simulink model "INtegrated_Simplified_Batteries_2"  (R2025a)
settings: Solver=ode113  StartTime=0.0  StopTime=20000  FixedStep=0.01  MaxStep=0.1  RelTol=1e-3
libraries: simulink x16, slpidlib x2, spsFirstOrderFilterLib x1
(part 3 of 3)

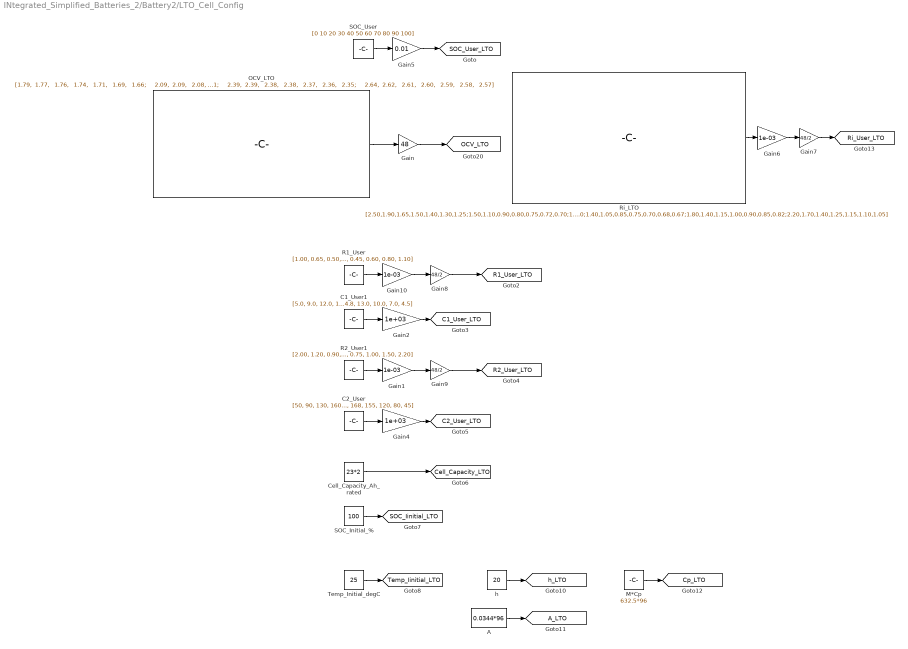
== system INtegrated_Simplified_Batteries_2/Battery2/LTO_Cell_Config ==
  A : Constant  Value=0.0344*96
  C1_User1 : Constant  Value=[5.0, 9.0, 12.0, 14.0, 14.8, 15.0, 14.8, 13.0, 10.0, 7.0, 4.5]
  C2_User : Constant  Value=[50, 90, 130, 160, 168, 170, 168, 155, 120, 80, 45]
  Cell_Capacity_Ah_rated : Constant  Value=23*2
  Gain : Gain  Gain=48
  Gain1 : Gain  Gain=1e-03
  Gain10 : Gain  Gain=1e-03
  Gain2 : Gain  Gain=1e+03
  Gain4 : Gain  Gain=1e+03
  Gain5 : Gain  Gain=0.01
  Gain6 : Gain  Gain=1e-03
  Gain7 : Gain  Gain=48/2
  Gain8 : Gain  Gain=48/2
  Gain9 : Gain  Gain=48/2
  M*Cp : Constant  Value=632.5*96
  OCV_LTO : Constant  Value=|
      | [1.79,  1.77,   1.76,   1.74,   1.71,   1.69,   1.66;
      |     2.09,  2.09,   2.08,   2.07,   2.06,   2.05,   2.04;
      |     2.19,  2.19,   2.18,   2.18,   2.17,   2.16,   2.15;
      |     2.23,  2.23,   2.23,   2.22,   2.22,   2.21,   2.21;
      |     2.25,  2.25,   2.25,   2.24,   2.24,   2.23,   2.23;
      |     2.28,  2.27,   2.27,   2.27,   2.26,   2.26,   2.25;
      |     2.30,  2.29,   2.29,   2.29,   2.28,   2.28,   2.27;
      |     2.32,  2.31,   2.31,   2.31,   2.30,   2.30,   2.29;
      |     2.34,  2.34,   2.34,   2.33,   2.33,   2.32,   2.31;
      |     2.39,  2.39,   2.38,   2.38,   2.37,   2.36,   2.35;
      |     2.64,  2.62,   2.61,   2.60,   2.59,   2.58,   2.57]
  R1_User : Constant  Value=[1.00, 0.65, 0.50, 0.40, 0.37, 0.35, 0.37, 0.45, 0.60, 0.80, 1.10]
  R2_User1 : Constant  Value=[2.00, 1.20, 0.90, 0.70, 0.62, 0.60, 0.62, 0.75, 1.00, 1.50, 2.20]
  Ri_LTO : Constant  Value=[2.50,1.90,1.65,1.50,1.40,1.30,1.25;1.50,1.10,0.90,0.80,0.75,0.72,0.70;1.25,0.95,0.75,0.65,0.60,0.58,0.57;1.10,0.80,0.60,0.52,0.48,0.47,0.46;1.05,0.75,0.55,0.48,0.45,0.44,0.43;1.00,0.70,0.52,0.45,0.42,0.41,0.40;1.05,0.75,0.55,0.48,0.45,0.44,0.43;1.15,0.85,0.65,0.57,0.53,0.51,0.50;1.40,1.05,0.85,0.75,0.70,0.68,0.67;1.80,1.40,1.15,1.00,0.90,0.85,0.82;2.20,1.70,1.40,1.25,1.15,1.10,1.05]
  SOC_Initial_% : Constant  Value=100
  SOC_User : Constant  Value=[0 10 20 30 40 50 60 70 80 90 100]
  Temp_Initial_degC : Constant  Value=25
  h : Constant  Value=20
  tag scope: A_LTO=global, C1_User_LTO=global, C2_User_LTO=global, Cell_Capacity_LTO=global, Cp_LTO=global, OCV_LTO=global, R1_User_LTO=global, R2_User_LTO=global, Ri_User_LTO=global, SOC_Iinitial_LTO=global, SOC_User_LTO=global, Temp_Iinitial_LTO=global, h_LTO=global
  wires:
  OCV_LTO/1 -> Gain/1
  SOC_User/1 -> Gain5/1
  R1_User/1 -> Gain10/1
  Gain10/1 -> Gain8/1
  C1_User1/1 -> Gain2/1
  Gain2/1 -> [C1_User_LTO]
  R2_User1/1 -> Gain1/1
  Gain1/1 -> Gain9/1
  Gain4/1 -> [C2_User_LTO]
  C2_User/1 -> Gain4/1
  Cell_Capacity_Ah_rated/1 -> [Cell_Capacity_LTO]
  SOC_Initial_%/1 -> [SOC_Iinitial_LTO]
  Gain5/1 -> [SOC_User_LTO]
  Temp_Initial_degC/1 -> [Temp_Iinitial_LTO]
  h/1 -> [h_LTO]
  A/1 -> [A_LTO]
  M*Cp/1 -> [Cp_LTO]
  Gain6/1 -> Gain7/1
  Ri_LTO/1 -> Gain6/1
  Gain/1 -> [OCV_LTO]
  Gain7/1 -> [Ri_User_LTO]
  Gain8/1 -> [R1_User_LTO]
  Gain9/1 -> [R2_User_LTO]

== system INtegrated_Simplified_Batteries_2/Battery2/Module2 ==
  Module_Current : Inport
  SubModule_1 : Subsystem
  Module_Voltage : Outport
  Module_avg_Temp : Outport  Port=2
  wires:
  SubModule_1/2(SubModule_avg_temp) -> Module_avg_Temp/1
  [Module_Current] -> SubModule_1/1(Module_Current)
  SubModule_1/1(SubModule_Voltage) -> Module_Voltage/1
  Module_Current/1 -> [Module_Current]

== system INtegrated_Simplified_Batteries_2/Battery2/SOCEstimator ==
  SOC_Initial : Inport
  Pack_Capacity : Inport  Port=2
  Current : Inport  Port=3
  SOCEstimator : Subsystem
  SOC : Outport
  wires:
  SOCEstimator/1(SOC) -> SOC/1
  SOC_Initial/1 -> SOCEstimator/1(SOC_Initial)
  Current/1 -> SOCEstimator/2(Current)
  Pack_Capacity/1 -> SOCEstimator/3(CellCapacity)

== system INtegrated_Simplified_Batteries_2/Observations/Battery1 Operation ==
  Battery1_Voltage : Inport
  Battery1_Current : Inport  Port=2
  Battery1_DischargeCurrLim : Inport  Port=3
  Battery1_ChargeCurrLim : Inport  Port=4
  Battery1_SOC : Inport  Port=5
  Battery1_Temperature : Inport  Port=6
  Battery1_Power : Inport  Port=7
  Battery1_Currents,Current_Limits&SOC : Scope  NumInputPorts=2
      settings: ActiveDisplayYMinimum=-282.10404867069661  ActiveDisplayYMaximum=307.35303677527855  DataLoggingVariableName=ScopeData2
  Battery1_Power&Temperature : Scope  NumInputPorts=2
      settings: ActiveDisplayYMinimum=22.791711351497295  ActiveDisplayYMaximum=44.874597836524366  DataLoggingVariableName=ScopeData3
  Battery1_Voltage&SOC : Scope  NumInputPorts=2
      settings: ActiveDisplayYMinimum=-1  ActiveDisplayYMaximum=1
  Mux : Mux  Inputs=3
  wires:
  Battery1_Voltage/1 -> Battery1_Voltage&SOC/1
  Battery1_SOC/1 -> Battery1_Voltage&SOC/2, Battery1_Currents,Current_Limits&SOC/2
  Mux/1 -> Battery1_Currents,Current_Limits&SOC/1
  Battery1_Current/1 -> Mux/1
  Battery1_DischargeCurrLim/1 -> Mux/2
  Battery1_ChargeCurrLim/1 -> Mux/3
  Battery1_Temperature/1 -> Battery1_Power&Temperature/1
  Battery1_Power/1 -> Battery1_Power&Temperature/2

== system INtegrated_Simplified_Batteries_2/Observations/Battery2 Operation ==
  Battery2_Voltage : Inport
  Battery2_Current : Inport  Port=2
  Battery2_DischargeCurrLim : Inport  Port=3
  Battery2_ChargeCurrLim : Inport  Port=4
  Battery2_SOC : Inport  Port=5
  Battery2_Temperature : Inport  Port=6
  Battery2_Power : Inport  Port=7
  Battery2_Currents,Current_Limits&SOC : Scope  NumInputPorts=2
      settings: ActiveDisplayYMinimum=-1129.3572740653772  ActiveDisplayYMaximum=1109.43488760312  DataLoggingVariableName=ScopeData2
  Battery2_Power&Temperature : Scope  NumInputPorts=2
      settings: ActiveDisplayYMinimum=22.713194675868088  ActiveDisplayYMaximum=45.581247917187227  DataLoggingVariableName=ScopeData3
  Battery2_Voltage&SOC : Scope  NumInputPorts=2
      settings: ActiveDisplayYMinimum=-1  ActiveDisplayYMaximum=1
  Mux : Mux  Inputs=3
  wires:
  Battery2_SOC/1 -> Battery2_Voltage&SOC/2, Battery2_Currents,Current_Limits&SOC/2
  Battery2_Voltage/1 -> Battery2_Voltage&SOC/1
  Battery2_ChargeCurrLim/1 -> Mux/3
  Battery2_Temperature/1 -> Battery2_Power&Temperature/1
  Battery2_Power/1 -> Battery2_Power&Temperature/2
  Battery2_DischargeCurrLim/1 -> Mux/2
  Battery2_Current/1 -> Mux/1
  Mux/1 -> Battery2_Currents,Current_Limits&SOC/1

== system INtegrated_Simplified_Batteries_2/Observations/DAB & Load Splitter Operation ==
  DAB_HighSideCurrentRef : Inport
  DAB_HighSideCurrent : Inport  Port=2
  DAB_PowerTransfer : Inport  Port=3
  Battery1_Current : Inport  Port=4
  Battery2_Current : Inport  Port=5
  Total_Current : Inport  Port=6
  Currents : Scope  NumInputPorts=2
      settings: ActiveDisplayYMinimum=-302.947845806585  ActiveDisplayYMaximum=379.10772170406915  DataLoggingVariableName=ScopeData6
  DAB_HighSideCurr : Scope  NumInputPorts=2
      settings: ActiveDisplayYMinimum=-1  ActiveDisplayYMaximum=1  DataLoggingVariableName=ScopeData4
  DAB_Power : Scope
      settings: ActiveDisplayYMinimum=-1  ActiveDisplayYMaximum=1  DataLoggingVariableName=ScopeData5
  Mux : Mux  Inputs=3
  wires:
  DAB_PowerTransfer/1 -> DAB_Power/1
  DAB_HighSideCurrent/1 -> DAB_HighSideCurr/2, Mux/2
  Battery1_Current/1 -> Mux/1
  Total_Current/1 -> Mux/3
  DAB_HighSideCurrentRef/1 -> DAB_HighSideCurr/1
  Mux/1 -> Currents/1
  Battery2_Current/1 -> Currents/2

== system INtegrated_Simplified_Batteries_2/Observations/System Operation ==
  RPM_request : Inport
  RPM_Actual : Inport  Port=2
  Vehicle_Speed : Inport  Port=3
  Electrical_Power : Inport  Port=4
  Mechanical_Power : Inport  Port=5
  System_Efficiency : Inport  Port=6
  Driveline_Torque_Request : Inport  Port=7
  Driveline_Torque : Inport  Port=8
  Avauilable_Motor_Torque : Inport  Port=9
  Vehicle_Acceleration : Inport  Port=10
  Motor_torque_Actual : Inport  Port=11
  Distance : Inport  Port=12
  Distance_Travelled : Display
  Mux : Mux  Inputs=2
  Mux1 : Mux  Inputs=2
  Mux2 : Mux  Inputs=2
  Power&Efficiency : Scope  NumInputPorts=2
      settings: ActiveDisplayYMinimum=-244.19267618677512  ActiveDisplayYMaximum=191.67830084577145  DataLoggingVariableName=ScopeData8
  RPM_Requested&Actual : Scope  NumInputPorts=2
      settings: ActiveDisplayYMinimum=-2374.9999999999995  ActiveDisplayYMaximum=21375  DataLoggingVariableName=ScopeData7
  Requested&Actual_Torques : Scope  NumInputPorts=3
      settings: ActiveDisplayYMinimum=-499.22287325827932  ActiveDisplayYMaximum=499.91365258425321  DataLoggingVariableName=ScopeData9
  VehicleSpeed&Acceleration : Scope  NumInputPorts=2
      settings: ActiveDisplayYMinimum=-1  ActiveDisplayYMaximum=1  DataLoggingVariableName=ScopeData10
  wires:
  RPM_request/1 -> Mux2/1
  RPM_Actual/1 -> Mux2/2
  Electrical_Power/1 -> Mux/1
  Mechanical_Power/1 -> Mux/2
  System_Efficiency/1 -> Power&Efficiency/2
  Mux/1 -> Power&Efficiency/1
  Mux1/1 -> Requested&Actual_Torques/1
  Driveline_Torque_Request/1 -> Mux1/1
  Driveline_Torque/1 -> Mux1/2
  Avauilable_Motor_Torque/1 -> Requested&Actual_Torques/2
  Vehicle_Speed/1 -> RPM_Requested&Actual/2, VehicleSpeed&Acceleration/1
  Mux2/1 -> RPM_Requested&Actual/1
  Vehicle_Acceleration/1 -> VehicleSpeed&Acceleration/2
  Motor_torque_Actual/1 -> Requested&Actual_Torques/3
  Distance/1 -> Distance_Travelled/1

== system INtegrated_Simplified_Batteries_2/Battery1/Module3/SubModule_1 ==
  Module_Current : Inport
  Cell1 : Subsystem
  SubModule_Voltage : Outport
  SubModule_avg_temp : Outport  Port=2
  wires:
  Cell1/2(Cell_temp) -> SubModule_avg_temp/1
  Cell1/1(Cell_Voltage) -> SubModule_Voltage/1
  [Cell_Current] -> Cell1/1(Cell_Current)
  Module_Current/1 -> [Cell_Current]

== system INtegrated_Simplified_Batteries_2/Battery1/SOCEstimator/SOCEstimator ==
  SOC_Initial : Inport
  Current : Inport  Port=2
  CellCapacity : Inport  Port=3
  Add1 : Sum  Inputs=+-
  Constant : Constant  Value=100  SampleTime=-1
  Constant1 : Constant  Value=3600  SampleTime=-1
  Delay : Delay  DelayLength=1  InitialConditionSource=Input port
      settings: InputPortMap=u0,p4
  Divide : Product  Inputs=*//
  Divide1 : Product  Inputs=*/
  Integrator : Integrator
  Rate Transition : RateTransition
  Saturation1 : Saturate  UpperLimit=1  LowerLimit=0
  SOC : Outport
  wires:
  Add1/1 -> Saturation1/1
  Constant/1 -> Divide1/2
  Divide1/1 -> Delay/2, Add1/1
  Divide/1 -> Add1/2
  Saturation1/1 -> Delay/1
  SOC_Initial/1 -> Divide1/1
  Current/1 -> Integrator/1
  Delay/1 -> Rate Transition/1
  CellCapacity/1 -> Divide/2
  Constant1/1 -> Divide/3
  Integrator/1 -> Divide/1
  Rate Transition/1 -> SOC/1

== system INtegrated_Simplified_Batteries_2/Battery2/Module2/SubModule_1 ==
  Module_Current : Inport
  Cell1 : Subsystem
  SubModule_Voltage : Outport
  SubModule_avg_temp : Outport  Port=2
  wires:
  Cell1/1(Cell_Voltage) -> SubModule_Voltage/1
  [Cell_Current] -> Cell1/1(Cell_Current)
  Module_Current/1 -> [Cell_Current]
  Cell1/2(Cell_temp) -> SubModule_avg_temp/1

== system INtegrated_Simplified_Batteries_2/Battery2/SOCEstimator/SOCEstimator ==
  SOC_Initial : Inport
  Current : Inport  Port=2
  CellCapacity : Inport  Port=3
  Add1 : Sum  Inputs=+-
  Constant : Constant  Value=100  SampleTime=-1
  Constant1 : Constant  Value=3600  SampleTime=-1
  Delay : Delay  DelayLength=1  InitialConditionSource=Input port
      settings: InputPortMap=u0,p4
  Divide : Product  Inputs=*//
  Divide1 : Product  Inputs=*/
  Integrator : Integrator
  Rate Transition : RateTransition
  Saturation1 : Saturate  UpperLimit=1  LowerLimit=0
  SOC : Outport
  wires:
  Add1/1 -> Saturation1/1
  Constant/1 -> Divide1/2
  Divide1/1 -> Delay/2, Add1/1
  Divide/1 -> Add1/2
  Saturation1/1 -> Delay/1
  SOC_Initial/1 -> Divide1/1
  Current/1 -> Integrator/1
  Delay/1 -> Rate Transition/1
  CellCapacity/1 -> Divide/2
  Constant1/1 -> Divide/3
  Integrator/1 -> Divide/1
  Rate Transition/1 -> SOC/1

== system INtegrated_Simplified_Batteries_2/Battery1/Module3/SubModule_1/Cell1 ==
  Cell_Current : Inport
  2RC : Subsystem
  Add : Sum  Inputs=---+
  Lookup Table Dynamic2 : simulink/Lookup Tables/Lookup Table Dynamic  LookUpMeth=Interpolation-Use End Values  OutDataType=fixdt('double')  OutScaling=[]  OutputDataTypeScalingMode=Specify via dialog  OutDataTypeStr=fixdt('double')  DoSatur=off
  Product : Product
  Redution_factor : Constant  Value=[0.8 0.85 0.88 0.95 1 0.98 0.95]
  SOCEstimator : Subsystem  TreatAsAtomicUnit=on
  SOC_Mapping : Subsystem
  Scope : Scope
      settings: DataLoggingSaveFormat=Array
  Scope1 : Scope
      settings: DataLoggingVariableName=ScopeData2  DataLoggingSaveFormat=Array
  Scope2 : Scope
      settings: DataLoggingSaveFormat=Array
  Subsystem : Subsystem
  Temp : Constant  Value=[0 10 20 30 40 50 60]
  Cell_Voltage : Outport
  Cell_temp : Outport  Port=2
  wires:
  Redution_factor/1 -> Lookup Table Dynamic2/3
  Temp/1 -> Lookup Table Dynamic2/2
  Lookup Table Dynamic2/1 -> Product/2
  Product/1 -> SOCEstimator/3(Cell_Capacity)
  Subsystem/1(Temp_Cell) -> Cell_temp/1, Lookup Table Dynamic2/1, SOC_Mapping/2(Cell_Temp), Scope1/1
  SOC_Mapping/6(OCV) -> Add/4
  [SOC_Iinitial] -> SOCEstimator/1(SOC_Initial)
  SOC_Mapping/4(R2) -> 2RC/5(R2)
  SOC_Mapping/5(C2) -> 2RC/6(C2)
  [Cell_Capacity] -> Product/1
  SOC_Mapping/2(R1) -> 2RC/3(R1)
  Cell_Current/1 -> SOCEstimator/2(Current), 2RC/1(Current), Subsystem/1(Cell_Current)
  2RC/3(Vi) -> Add/3
  2RC/1(V1) -> Add/1
  SOC_Mapping/1(Ri) -> 2RC/2(Ri), Subsystem/2(Ri)
  Add/1 -> Cell_Voltage/1, Scope2/1
  SOCEstimator/1(SOC) -> Scope/1, SOC_Mapping/1(SOC)
  SOC_Mapping/3(C1) -> 2RC/4(C1)
  2RC/2(V2) -> Add/2

== system INtegrated_Simplified_Batteries_2/Battery2/Module2/SubModule_1/Cell1 ==
  Cell_Current : Inport
  2RC : Subsystem
  Add : Sum  Inputs=---+
  Lookup Table Dynamic2 : simulink/Lookup Tables/Lookup Table Dynamic  LookUpMeth=Interpolation-Use End Values  OutDataType=fixdt('double')  OutScaling=[]  OutputDataTypeScalingMode=Specify via dialog  OutDataTypeStr=fixdt('double')  DoSatur=off
  Product : Product
  Redution_factor : Constant  Value=[0.8 0.85 0.88 0.95 1 0.98 0.95]
  SOCEstimator : Subsystem  TreatAsAtomicUnit=on
  SOC_Mapping : Subsystem
  Scope : Scope
      settings: DataLoggingSaveFormat=Array
  Scope1 : Scope
      settings: DataLoggingVariableName=ScopeData2  DataLoggingSaveFormat=Array
  Scope2 : Scope
      settings: DataLoggingSaveFormat=Array
  Subsystem : Subsystem
  Temp : Constant  Value=[0 10 20 30 40 50 60]
  Cell_Voltage : Outport
  Cell_temp : Outport  Port=2
  wires:
  Redution_factor/1 -> Lookup Table Dynamic2/3
  Temp/1 -> Lookup Table Dynamic2/2
  Lookup Table Dynamic2/1 -> Product/2
  Product/1 -> SOCEstimator/3(Cell_Capacity)
  Subsystem/1(Temp_Cell) -> Cell_temp/1, Lookup Table Dynamic2/1, SOC_Mapping/2(Cell_Temp), Scope1/1
  SOC_Mapping/6(OCV) -> Add/4
  [SOC_Iinitial_LTO] -> SOCEstimator/1(SOC_Initial)
  SOC_Mapping/4(R2) -> 2RC/5(R2)
  SOC_Mapping/5(C2) -> 2RC/6(C2)
  [Cell_Capacity_LTO] -> Product/1
  SOC_Mapping/2(R1) -> 2RC/3(R1)
  Cell_Current/1 -> SOCEstimator/2(Current), 2RC/1(Current), Subsystem/1(Cell_Current)
  2RC/3(Vi) -> Add/3
  2RC/1(V1) -> Add/1
  SOC_Mapping/1(Ri) -> 2RC/2(Ri), Subsystem/2(Ri)
  Add/1 -> Cell_Voltage/1, Scope2/1
  SOCEstimator/1(SOC) -> Scope/1, SOC_Mapping/1(SOC)
  SOC_Mapping/3(C1) -> 2RC/4(C1)
  2RC/2(V2) -> Add/2

== system INtegrated_Simplified_Batteries_2/Battery1/Module3/SubModule_1/Cell1/2RC ==
  Current : Inport
  Ri : Inport  Port=2
  R1 : Inport  Port=3
  C1 : Inport  Port=4
  R2 : Inport  Port=5
  C2 : Inport  Port=6
  RC1 : Subsystem
  RC2 : Subsystem
  Rint : Subsystem
  V1 : Outport
  V2 : Outport  Port=2
  Vi : Outport  Port=3
  wires:
  Ri/1 -> Rint/2(R)
  C2/1 -> RC2/3(C)
  RC2/1(V) -> V2/1
  RC1/1(V) -> V1/1
  R2/1 -> RC2/2(R)
  C1/1 -> RC1/3(C)
  Rint/1(V) -> Vi/1
  R1/1 -> RC1/2(R)
  Current/1 -> RC2/1(Current), RC1/1(Current), Rint/1(Current)

== system INtegrated_Simplified_Batteries_2/Battery1/Module3/SubModule_1/Cell1/SOCEstimator ==
  SOC_Initial : Inport
  Current : Inport  Port=2
  Cell_Capacity : Inport  Port=3
  SOCEstimator : Subsystem
  SOC : Outport
  wires:
  Cell_Capacity/1 -> SOCEstimator/3(CellCapacity)
  Current/1 -> SOCEstimator/2(Current)
  SOC_Initial/1 -> SOCEstimator/1(SOC_Initial)
  SOCEstimator/1(SOC) -> SOC/1

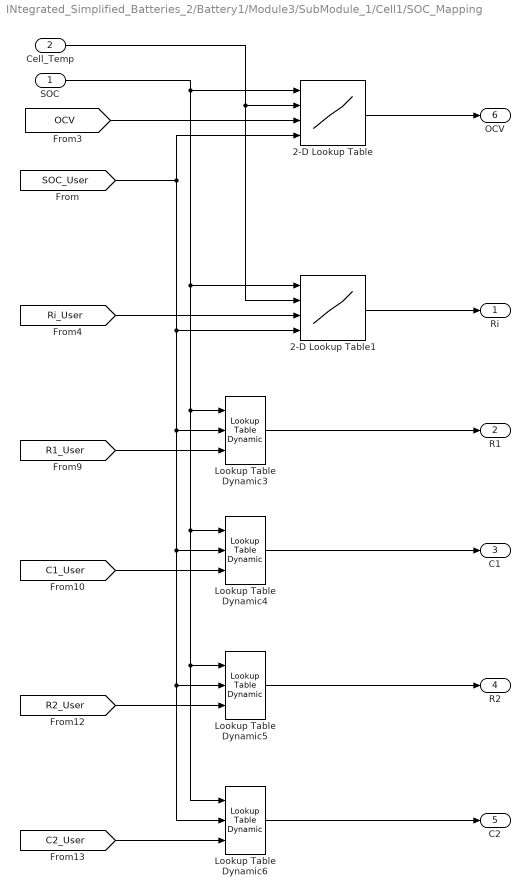
== system INtegrated_Simplified_Batteries_2/Battery1/Module3/SubModule_1/Cell1/SOC_Mapping ==
  SOC : Inport
  Cell_Temp : Inport  Port=2
  2-D Lookup Table : Lookup_n-D  LookupTableObject=''  BreakpointsForDimension1Source=Input port  BreakpointsForDimension1=[0 0.1 0.2 0.3 0.4 0.5 0.6 0.7 0.8 0.9 1]  BreakpointsForDimension2=[0 10 20 30 40 50 60]  BreakpointsForDimension1FirstPoint=10  BreakpointsForDimension2FirstPoint=10  BreakpointsForDimension1Spacing=12  BreakpointsForDimension2Spacing=12  IndexSearchMethod=Evenly spaced points  TableSource=Input port  Table=|  InterpMethod=Akima spline  DiagnosticForOutOfRangeInput=Error  InternalRulePriority=Speed  RndMeth=Simplest
      | [
      |     2.954364, 3.109857, 3.273534, 3.3066, 3.34,    3.3734,  3.20473;
      |     3.122427, 3.286765, 3.459753, 3.4947, 3.53,    3.5653,  3.387035;
      |     3.175499, 3.342631, 3.518559, 3.5541, 3.59,    3.6259,  3.444605;
      |     3.210881, 3.379875, 3.557763, 3.5937, 3.63,    3.6663,  3.482985;
      |     3.237417, 3.407808, 3.587166, 3.6234, 3.66,    3.6966,  3.511777;
      |     3.272799, 3.445052, 3.62637,  3.663,  3.7,     3.737,   3.55015;
      |     3.317026, 3.491066, 3.675375, 3.7125, 3.75,    3.7875,  3.598125;
      |     3.387789, 3.566094, 3.753783, 3.7917, 3.83,    3.8683,  3.674885;
      |     3.467398, 3.649892, 3.841992, 3.8808, 3.92,    3.9592,  3.76124;
      |     3.564697, 3.752313, 3.949803, 3.9897, 4.03,    4.0703,  3.866785;
      |     3.653151, 3.845422, 4.047813, 4.0887, 4.13,    4.1713,  3.962735
      | ]
      settings: InputPortMap=u0,u1,p221,p5
  2-D Lookup Table1 : Lookup_n-D  LookupTableObject=''  BreakpointsForDimension1Source=Input port  BreakpointsForDimension1=[0 0.1 0.2 0.3 0.4 0.5 0.6 0.7 0.8 0.9 1]  BreakpointsForDimension2=[0 10 20 30 40 50 60]  BreakpointsForDimension1FirstPoint=10  BreakpointsForDimension2FirstPoint=10  BreakpointsForDimension1Spacing=12  BreakpointsForDimension2Spacing=12  IndexSearchMethod=Evenly spaced points  TableSource=Input port  Table=|  InterpMethod=Akima spline  DiagnosticForOutOfRangeInput=Error  InternalRulePriority=Speed  RndMeth=Simplest
      | [
      |     2.954364, 3.109857, 3.273534, 3.3066, 3.34,    3.3734,  3.20473;
      |     3.122427, 3.286765, 3.459753, 3.4947, 3.53,    3.5653,  3.387035;
      |     3.175499, 3.342631, 3.518559, 3.5541, 3.59,    3.6259,  3.444605;
      |     3.210881, 3.379875, 3.557763, 3.5937, 3.63,    3.6663,  3.482985;
      |     3.237417, 3.407808, 3.587166, 3.6234, 3.66,    3.6966,  3.511777;
      |     3.272799, 3.445052, 3.62637,  3.663,  3.7,     3.737,   3.55015;
      |     3.317026, 3.491066, 3.675375, 3.7125, 3.75,    3.7875,  3.598125;
      |     3.387789, 3.566094, 3.753783, 3.7917, 3.83,    3.8683,  3.674885;
      |     3.467398, 3.649892, 3.841992, 3.8808, 3.92,    3.9592,  3.76124;
      |     3.564697, 3.752313, 3.949803, 3.9897, 4.03,    4.0703,  3.866785;
      |     3.653151, 3.845422, 4.047813, 4.0887, 4.13,    4.1713,  3.962735
      | ]
      settings: InputPortMap=u0,u1,p221,p5
  Lookup Table Dynamic{3..6} (4 alike) : simulink/Lookup Tables/Lookup Table Dynamic  LookUpMeth=Interpolation-Use End Values  OutDataType=fixdt('double')  OutScaling=[]  OutputDataTypeScalingMode=Specify via dialog  OutDataTypeStr=fixdt('double')  DoSatur=off
  Ri : Outport
  R1 : Outport  Port=2
  C1 : Outport  Port=3
  R2 : Outport  Port=4
  C2 : Outport  Port=5
  OCV : Outport  Port=6
  wires:
  Cell_Temp/1 -> 2-D Lookup Table/2, 2-D Lookup Table1/2
  Lookup Table Dynamic6/1 -> C2/1
  [C2_User] -> Lookup Table Dynamic6/3
  Lookup Table Dynamic5/1 -> R2/1
  [R2_User] -> Lookup Table Dynamic5/3
  Lookup Table Dynamic4/1 -> C1/1
  [C1_User] -> Lookup Table Dynamic4/3
  Lookup Table Dynamic3/1 -> R1/1
  [R1_User] -> Lookup Table Dynamic3/3
  2-D Lookup Table1/1 -> Ri/1
  [Ri_User] -> 2-D Lookup Table1/3
  2-D Lookup Table/1 -> OCV/1
  [OCV] -> 2-D Lookup Table/3
  [SOC_User] -> 2-D Lookup Table1/4, Lookup Table Dynamic3/2, Lookup Table Dynamic4/2, Lookup Table Dynamic5/2, Lookup Table Dynamic6/2, 2-D Lookup Table/4
  SOC/1 -> 2-D Lookup Table/1, 2-D Lookup Table1/1, Lookup Table Dynamic4/1, Lookup Table Dynamic5/1, Lookup Table Dynamic6/1, Lookup Table Dynamic3/1

== system INtegrated_Simplified_Batteries_2/Battery1/Module3/SubModule_1/Cell1/Subsystem ==
  Cell_Current : Inport
  Ri : Inport  Port=2
  Add : Sum  Inputs=+-
  Add1 : Sum  Inputs=-+
  Delay : Delay  DelayLength=1  InitialConditionSource=Input port
      settings: InputPortMap=u0,p4
  Divide : Product  Inputs=*/
  From3 : From  TagVisibility=global
  Integrator : Integrator  InitialConditionSource=external
  Product{,1..3} (4 alike) : Product
  Temp_Cell : Outport
  wires:
  [Cp] -> Divide/2
  Delay/1 -> Add/1
  [Temp_Iinitial] -> Integrator/2, Delay/2
  Divide/1 -> Integrator/1
  Add1/1 -> Divide/1
  Product1/1 -> Add1/2
  Product3/1 -> Add1/1
  Add/1 -> Product3/1
  [Temp_ambient] -> Add/2
  Product2/1 -> Product3/2
  From3/1 -> Product2/2
  [h] -> Product2/1
  Ri/1 -> Product1/2
  Product/1 -> Product1/1
  Cell_Current/1 -> Product/1, Product/2
  Integrator/1 -> Delay/1, Temp_Cell/1

== system INtegrated_Simplified_Batteries_2/Battery2/Module2/SubModule_1/Cell1/2RC ==
  Current : Inport
  Ri : Inport  Port=2
  R1 : Inport  Port=3
  C1 : Inport  Port=4
  R2 : Inport  Port=5
  C2 : Inport  Port=6
  RC1 : Subsystem
  RC2 : Subsystem
  Rint : Subsystem
  V1 : Outport
  V2 : Outport  Port=2
  Vi : Outport  Port=3
  wires:
  Ri/1 -> Rint/2(R)
  C2/1 -> RC2/3(C)
  RC2/1(V) -> V2/1
  RC1/1(V) -> V1/1
  R2/1 -> RC2/2(R)
  C1/1 -> RC1/3(C)
  Rint/1(V) -> Vi/1
  R1/1 -> RC1/2(R)
  Current/1 -> RC2/1(Current), RC1/1(Current), Rint/1(Current)

== system INtegrated_Simplified_Batteries_2/Battery2/Module2/SubModule_1/Cell1/SOCEstimator ==
  SOC_Initial : Inport
  Current : Inport  Port=2
  Cell_Capacity : Inport  Port=3
  SOCEstimator : Subsystem
  SOC : Outport
  wires:
  Cell_Capacity/1 -> SOCEstimator/3(CellCapacity)
  Current/1 -> SOCEstimator/2(Current)
  SOC_Initial/1 -> SOCEstimator/1(SOC_Initial)
  SOCEstimator/1(SOC) -> SOC/1

== system INtegrated_Simplified_Batteries_2/Battery2/Module2/SubModule_1/Cell1/SOC_Mapping ==
  SOC : Inport
  Cell_Temp : Inport  Port=2
  2-D Lookup Table : Lookup_n-D  LookupTableObject=''  BreakpointsForDimension1Source=Input port  BreakpointsForDimension1=[0 0.1 0.2 0.3 0.4 0.5 0.6 0.7 0.8 0.9 1]  BreakpointsForDimension2=[0 10 20 30 40 50 60]  BreakpointsForDimension1FirstPoint=10  BreakpointsForDimension2FirstPoint=10  BreakpointsForDimension1Spacing=12  BreakpointsForDimension2Spacing=12  IndexSearchMethod=Evenly spaced points  TableSource=Input port  Table=|  InterpMethod=Akima spline  DiagnosticForOutOfRangeInput=Error  InternalRulePriority=Speed  RndMeth=Simplest
      | [
      |     2.954364, 3.109857, 3.273534, 3.3066, 3.34,    3.3734,  3.20473;
      |     3.122427, 3.286765, 3.459753, 3.4947, 3.53,    3.5653,  3.387035;
      |     3.175499, 3.342631, 3.518559, 3.5541, 3.59,    3.6259,  3.444605;
      |     3.210881, 3.379875, 3.557763, 3.5937, 3.63,    3.6663,  3.482985;
      |     3.237417, 3.407808, 3.587166, 3.6234, 3.66,    3.6966,  3.511777;
      |     3.272799, 3.445052, 3.62637,  3.663,  3.7,     3.737,   3.55015;
      |     3.317026, 3.491066, 3.675375, 3.7125, 3.75,    3.7875,  3.598125;
      |     3.387789, 3.566094, 3.753783, 3.7917, 3.83,    3.8683,  3.674885;
      |     3.467398, 3.649892, 3.841992, 3.8808, 3.92,    3.9592,  3.76124;
      |     3.564697, 3.752313, 3.949803, 3.9897, 4.03,    4.0703,  3.866785;
      |     3.653151, 3.845422, 4.047813, 4.0887, 4.13,    4.1713,  3.962735
      | ]
      settings: InputPortMap=u0,u1,p221,p5
  2-D Lookup Table1 : Lookup_n-D  LookupTableObject=''  BreakpointsForDimension1Source=Input port  BreakpointsForDimension1=[0 0.1 0.2 0.3 0.4 0.5 0.6 0.7 0.8 0.9 1]  BreakpointsForDimension2=[0 10 20 30 40 50 60]  BreakpointsForDimension1FirstPoint=10  BreakpointsForDimension2FirstPoint=10  BreakpointsForDimension1Spacing=12  BreakpointsForDimension2Spacing=12  IndexSearchMethod=Evenly spaced points  TableSource=Input port  Table=|  InterpMethod=Akima spline  InternalRulePriority=Speed  RndMeth=Simplest
      | [
      |     2.954364, 3.109857, 3.273534, 3.3066, 3.34,    3.3734,  3.20473;
      |     3.122427, 3.286765, 3.459753, 3.4947, 3.53,    3.5653,  3.387035;
      |     3.175499, 3.342631, 3.518559, 3.5541, 3.59,    3.6259,  3.444605;
      |     3.210881, 3.379875, 3.557763, 3.5937, 3.63,    3.6663,  3.482985;
      |     3.237417, 3.407808, 3.587166, 3.6234, 3.66,    3.6966,  3.511777;
      |     3.272799, 3.445052, 3.62637,  3.663,  3.7,     3.737,   3.55015;
      |     3.317026, 3.491066, 3.675375, 3.7125, 3.75,    3.7875,  3.598125;
      |     3.387789, 3.566094, 3.753783, 3.7917, 3.83,    3.8683,  3.674885;
      |     3.467398, 3.649892, 3.841992, 3.8808, 3.92,    3.9592,  3.76124;
      |     3.564697, 3.752313, 3.949803, 3.9897, 4.03,    4.0703,  3.866785;
      |     3.653151, 3.845422, 4.047813, 4.0887, 4.13,    4.1713,  3.962735
      | ]
      settings: InputPortMap=u0,u1,p221,p5
  Lookup Table Dynamic{3..6} (4 alike) : simulink/Lookup Tables/Lookup Table Dynamic  LookUpMeth=Interpolation-Use End Values  OutDataType=fixdt('double')  OutScaling=[]  OutputDataTypeScalingMode=Specify via dialog  OutDataTypeStr=fixdt('double')  DoSatur=off
  Ri : Outport
  R1 : Outport  Port=2
  C1 : Outport  Port=3
  R2 : Outport  Port=4
  C2 : Outport  Port=5
  OCV : Outport  Port=6
  wires:
  Cell_Temp/1 -> 2-D Lookup Table/2, 2-D Lookup Table1/2
  Lookup Table Dynamic6/1 -> C2/1
  [C2_User_LTO] -> Lookup Table Dynamic6/3
  Lookup Table Dynamic5/1 -> R2/1
  [R2_User_LTO] -> Lookup Table Dynamic5/3
  Lookup Table Dynamic4/1 -> C1/1
  [C1_User_LTO] -> Lookup Table Dynamic4/3
  Lookup Table Dynamic3/1 -> R1/1
  [R1_User_LTO] -> Lookup Table Dynamic3/3
  2-D Lookup Table1/1 -> Ri/1
  [Ri_User_LTO] -> 2-D Lookup Table1/3
  2-D Lookup Table/1 -> OCV/1
  [OCV_LTO] -> 2-D Lookup Table/3
  [SOC_User_LTO] -> 2-D Lookup Table1/4, Lookup Table Dynamic3/2, Lookup Table Dynamic4/2, Lookup Table Dynamic5/2, Lookup Table Dynamic6/2, 2-D Lookup Table/4
  SOC/1 -> 2-D Lookup Table/1, 2-D Lookup Table1/1, Lookup Table Dynamic4/1, Lookup Table Dynamic5/1, Lookup Table Dynamic6/1, Lookup Table Dynamic3/1

== system INtegrated_Simplified_Batteries_2/Battery2/Module2/SubModule_1/Cell1/Subsystem ==
  Cell_Current : Inport
  Ri : Inport  Port=2
  Add : Sum  Inputs=+-
  Add1 : Sum  Inputs=-+
  Delay : Delay  DelayLength=1  InitialConditionSource=Input port
      settings: InputPortMap=u0,p4
  Divide : Product  Inputs=*/
  Integrator : Integrator  InitialConditionSource=external
  Product{,1..3} (4 alike) : Product
  Temp_Cell : Outport
  wires:
  [Cp_LTO] -> Divide/2
  Delay/1 -> Add/1
  [Temp_Iinitial_LTO] -> Integrator/2, Delay/2
  Divide/1 -> Integrator/1
  Add1/1 -> Divide/1
  Product1/1 -> Add1/2
  Product3/1 -> Add1/1
  Add/1 -> Product3/1
  [Temp_ambient] -> Add/2
  Product2/1 -> Product3/2
  [A_LTO] -> Product2/2
  [h_LTO] -> Product2/1
  Ri/1 -> Product1/2
  Product/1 -> Product1/1
  Cell_Current/1 -> Product/1, Product/2
  Integrator/1 -> Delay/1, Temp_Cell/1

== system INtegrated_Simplified_Batteries_2/Battery1/Module3/SubModule_1/Cell1/2RC/RC1 ==
  Current : Inport
  R : Inport  Port=2
  C : Inport  Port=3
  2 : Constant
  Add : Sum
  Divide : Product  Inputs=*/
  Divide1 : Product  Inputs=*/
  Divide2 : Product  Inputs=/*
  Divide3 : Product  Inputs=**
  Integrator1 : Integrator
  Integrator2 : Integrator
  V : Outport
  wires:
  2/1 -> Divide2/2
  Integrator2/1 -> Add/2
  Divide3/1 -> V/1
  Current/1 -> Divide3/1
  Divide/1 -> Divide3/2
  Divide2/1 -> Integrator2/1
  R/1 -> Divide1/1, Add/1
  Add/1 -> Divide/2
  Divide1/1 -> Integrator1/1
  Integrator1/1 -> Divide/1
  C/1 -> Divide1/2, Divide2/1

== system INtegrated_Simplified_Batteries_2/Battery1/Module3/SubModule_1/Cell1/2RC/RC2 ==
  Current : Inport
  R : Inport  Port=2
  C : Inport  Port=3
  2 : Constant
  Add : Sum
  Divide : Product  Inputs=*/
  Divide1 : Product  Inputs=*/
  Divide2 : Product  Inputs=/*
  Divide3 : Product  Inputs=**
  Integrator1 : Integrator
  Integrator2 : Integrator
  V : Outport
  wires:
  C/1 -> Divide2/1, Divide1/2
  Integrator1/1 -> Divide/1
  Divide1/1 -> Integrator1/1
  Add/1 -> Divide/2
  R/1 -> Add/1, Divide1/1
  Divide2/1 -> Integrator2/1
  Divide/1 -> Divide3/2
  Current/1 -> Divide3/1
  Divide3/1 -> V/1
  Integrator2/1 -> Add/2
  2/1 -> Divide2/2

== system INtegrated_Simplified_Batteries_2/Battery1/Module3/SubModule_1/Cell1/2RC/Rint ==
  Current : Inport
  R : Inport  Port=2
  Divide3 : Product  Inputs=**
  V : Outport
  wires:
  Divide3/1 -> V/1
  Current/1 -> Divide3/1
  R/1 -> Divide3/2

== system INtegrated_Simplified_Batteries_2/Battery1/Module3/SubModule_1/Cell1/SOCEstimator/SOCEstimator ==
  SOC_Initial : Inport
  Current : Inport  Port=2
  CellCapacity : Inport  Port=3
  Add1 : Sum  Inputs=+-
  Constant : Constant  Value=100  SampleTime=-1
  Constant1 : Constant  Value=3600  SampleTime=-1
  Delay : Delay  DelayLength=1  InitialConditionSource=Input port
      settings: InputPortMap=u0,p4
  Divide : Product  Inputs=*//
  Divide1 : Product  Inputs=*/
  Integrator : Integrator
  Saturation1 : Saturate  UpperLimit=1  LowerLimit=0
  SOC : Outport
  wires:
  Integrator/1 -> Divide/1
  Constant1/1 -> Divide/3
  CellCapacity/1 -> Divide/2
  Delay/1 -> SOC/1
  Current/1 -> Integrator/1
  SOC_Initial/1 -> Divide1/1
  Saturation1/1 -> Delay/1
  Divide/1 -> Add1/2
  Divide1/1 -> Add1/1, Delay/2
  Constant/1 -> Divide1/2
  Add1/1 -> Saturation1/1

== system INtegrated_Simplified_Batteries_2/Battery2/Module2/SubModule_1/Cell1/2RC/RC1 ==
  Current : Inport
  R : Inport  Port=2
  C : Inport  Port=3
  2 : Constant
  Add : Sum
  Divide : Product  Inputs=*/
  Divide1 : Product  Inputs=*/
  Divide2 : Product  Inputs=/*
  Divide3 : Product  Inputs=**
  Integrator1 : Integrator
  Integrator2 : Integrator
  V : Outport
  wires:
  2/1 -> Divide2/2
  Integrator2/1 -> Add/2
  Divide3/1 -> V/1
  Current/1 -> Divide3/1
  Divide/1 -> Divide3/2
  Divide2/1 -> Integrator2/1
  R/1 -> Divide1/1, Add/1
  Add/1 -> Divide/2
  Divide1/1 -> Integrator1/1
  Integrator1/1 -> Divide/1
  C/1 -> Divide1/2, Divide2/1

== system INtegrated_Simplified_Batteries_2/Battery2/Module2/SubModule_1/Cell1/2RC/RC2 ==
  Current : Inport
  R : Inport  Port=2
  C : Inport  Port=3
  2 : Constant
  Add : Sum
  Divide : Product  Inputs=*/
  Divide1 : Product  Inputs=*/
  Divide2 : Product  Inputs=/*
  Divide3 : Product  Inputs=**
  Integrator1 : Integrator
  Integrator2 : Integrator
  V : Outport
  wires:
  C/1 -> Divide2/1, Divide1/2
  Integrator1/1 -> Divide/1
  Divide1/1 -> Integrator1/1
  Add/1 -> Divide/2
  R/1 -> Add/1, Divide1/1
  Divide2/1 -> Integrator2/1
  Divide/1 -> Divide3/2
  Current/1 -> Divide3/1
  Divide3/1 -> V/1
  Integrator2/1 -> Add/2
  2/1 -> Divide2/2

== system INtegrated_Simplified_Batteries_2/Battery2/Module2/SubModule_1/Cell1/2RC/Rint ==
  Current : Inport
  R : Inport  Port=2
  Divide3 : Product  Inputs=**
  V : Outport
  wires:
  Divide3/1 -> V/1
  Current/1 -> Divide3/1
  R/1 -> Divide3/2

== system INtegrated_Simplified_Batteries_2/Battery2/Module2/SubModule_1/Cell1/SOCEstimator/SOCEstimator ==
  SOC_Initial : Inport
  Current : Inport  Port=2
  CellCapacity : Inport  Port=3
  Add1 : Sum  Inputs=+-
  Constant : Constant  Value=100  SampleTime=-1
  Constant1 : Constant  Value=3600  SampleTime=-1
  Delay : Delay  DelayLength=1  InitialConditionSource=Input port
      settings: InputPortMap=u0,p4
  Divide : Product  Inputs=*//
  Divide1 : Product  Inputs=*/
  Integrator : Integrator
  Saturation1 : Saturate  UpperLimit=1  LowerLimit=0
  SOC : Outport
  wires:
  Integrator/1 -> Divide/1
  Constant1/1 -> Divide/3
  CellCapacity/1 -> Divide/2
  Delay/1 -> SOC/1
  Current/1 -> Integrator/1
  SOC_Initial/1 -> Divide1/1
  Saturation1/1 -> Delay/1
  Divide/1 -> Add1/2
  Divide1/1 -> Add1/1, Delay/2
  Constant/1 -> Divide1/2
  Add1/1 -> Saturation1/1

== matlab function INtegrated_Simplified_Batteries_2/Load Splitter/Load_Split ==
  data: I_Load input; I_Battery1 output; I_Battery2 output; factor input; Max_I_Battery1 input; I_Battery2_act input; Max_I_Battery2 input
function [I_Battery1, I_Battery2] = Load_Split(I_Load,factor,Max_I_Battery1,I_Battery2_act, Max_I_Battery2)
I_Battery1 = 0;
I_Battery2 = 0;
if abs(I_Load) < factor*Max_I_Battery1
    I_Battery1 = I_Load;
    I_Battery2 = 0;
elseif I_Load > 0
    if (I_Load - factor*Max_I_Battery1) < Max_I_Battery2
        I_Battery2 = I_Load - factor*Max_I_Battery1;
    %I_Battery1 = factor*Max_I_Battery1;
    else
        I_Battery2 = Max_I_Battery2;
    end
    I_Battery1 = I_Load - I_Battery2_act;
elseif I_Load < 0
    if abs(I_Load + factor*Max_I_Battery1) > Max_I_Battery2
        I_Battery2 = I_Load + factor*Max_I_Battery1;
    %I_Battery1 = -factor*Max_I_Battery1;
    else
        I_Battery2 = -1*Max_I_Battery2;
    end
    I_Battery1 = I_Load - I_Battery2_act;
end

== matlab function INtegrated_Simplified_Batteries_2/DAB_Converter/DAB_Power_Eqn ==
  data: V1 input; P output; V2 input; phi input; n input; f input; L input
function P = dab_power(V1, V2, phi, n, f, L)   % This is a more explicit version to satisfy the code analyzer. \n   % Define a constant for pi. \n   
PI_CONST = 3.1415926535;  % Calculate the main gain term. \n   
K = (n * V1 * V2) / (2 * PI_CONST * f * L); % Calculate the term dependent on the phase shift. \n   
phi_term = phi * (1 - abs(phi)/PI_CONST); % Assign the final output. \n  
P = K * phi_term;

== matlab function INtegrated_Simplified_Batteries_2/Current Calculator/MATLAB Function ==
  data: Torque input; Quadrant output; Speed input
function Quadrant = Quadrant_Selector(Torque,Speed)
if (Torque*Speed) < 0
    Quadrant = 0;
else
    Quadrant = 1;
end
